simulink model "Topic6"  (R2018b)
settings: Solver=FixedStepDiscrete  StartTime=0.0  StopTime=10.0  FixedStep=0.2  RelTol=1e-3
undefined symbols (not defined in the file or in its folder): ErrorStatus
libraries: simulink x2
settings Model: Creator=ayamu  LastModifiedBy=ayamu

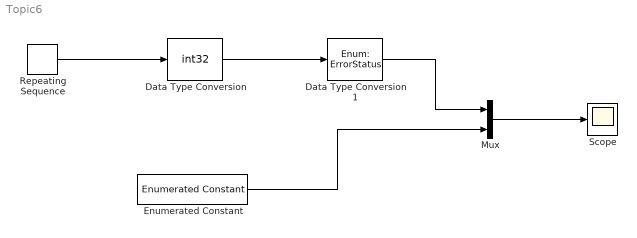
== system Topic6 ==
  Data Type Conversion : DataTypeConversion  OutDataTypeStr=int32
  Data Type Conversion1 : DataTypeConversion  OutDataTypeStr=Enum: ErrorStatus
  Enumerated Constant : simulink/Sources/Enumerated Constant  OutDataTypeStr=Enum: ErrorStatus  Value=ErrorStatus.Rcc_enuOK  SampleTime=inf
      settings: SourceProductName=Simulink
  Mux : Mux  Inputs=2
  Repeating Sequence : simulink/Sources/Repeating Sequence  rep_seq_t=[0 1 2 3 4]  rep_seq_y=[0 1 2 2 1]
  Scope : Scope
  wires:
  Enumerated Constant/1 -> Mux/2
  Repeating Sequence/1 -> Data Type Conversion/1
  Data Type Conversion1/1 -> Mux/1
  Data Type Conversion/1 -> Data Type Conversion1/1
  Mux/1 -> Scope/1
